simulink library "normalForce_ul"  (R2020a)
settings: Solver=VariableStepAuto  StartTime=0.0  StopTime=10.0  RelTol=1e-3
undefined symbols (not defined in the file): Veh
libraries: simulink x2, vrlib x1
settings Model: Creator=John Jr  LastModifiedBy=John Jr

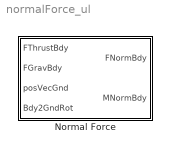
== system normalForce_ul ==
  Normal Force : Subsystem
      mask Display:
      | patch([0 1 1 0], [0 0 1 1],[.8 1 1])
      | 
      | port_label('input',1,'\fontname{Cambria Math}FThrustBdy','texmode','on')
      | port_label('input',2,'\fontname{Cambria Math}FGravBdy','texmode','on')
      | port_label('input',3,'\fontname{Cambria Math}posVecGnd','texmode','on')
      | port_label('input',4,'\fontname{Cambria Math}Bdy2GndRot','texmode','on')
      | 
      | port_label('output',1,'\fontname{Cambria Math}FNormBdy','texmode','on')
      | port_label('output',2,'\fontname{Cambria Math}MNormBdy','texmode','on')

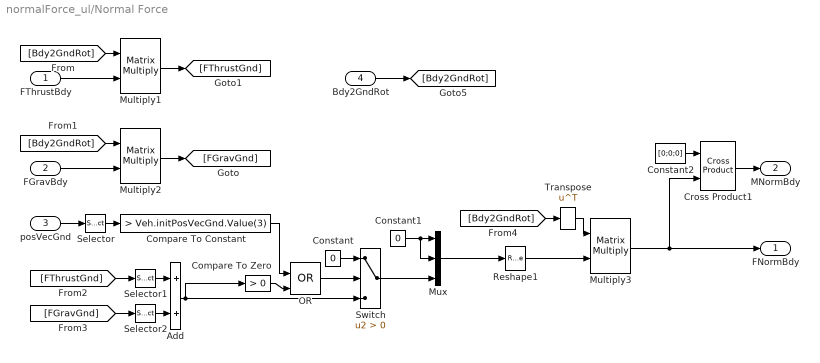
== system normalForce_ul/Normal Force ==
  FThrustBdy : Inport
  FGravBdy : Inport  Port=2
  posVecGnd : Inport  Port=3
  Bdy2GndRot : Inport  Port=4
  Add : Sum
  Compare To Constant : simulink/Logic and Bit Operations/Compare To Constant  relop=>  const=Veh.initPosVecGnd.Value(3)  OutDataTypeStr=boolean
  Compare To Zero : simulink/Logic and Bit Operations/Compare To Zero  relop=>  OutDataTypeStr=boolean
  Constant : Constant  Value=0
  Constant1 : Constant  Value=0
  Constant2 : Constant  Value=[0;0;0]
  Cross Product1 : vrlib/Utilities/Cross Product
  Multiply1 : Product  Multiplication=Matrix(*)
  Multiply2 : Product  Multiplication=Matrix(*)
  Multiply3 : Product  Multiplication=Matrix(*)
  Mux : Mux  Inputs=3
  OR : Logic  Operator=OR  IconShape=distinctive  AllPortsSameDT=off  OutDataTypeStr=boolean
  Reshape1 : Reshape  OutputDimensionality=Column vector (2-D)
  Selector : Selector  InputPortWidth=3  IndexOptions=Index vector (dialog)  Indices=3  OutputSizes=1
  Selector1 : Selector  InputPortWidth=3  IndexOptions=Index vector (dialog)  Indices=3  OutputSizes=1
  Selector2 : Selector  InputPortWidth=3  IndexOptions=Index vector (dialog)  Indices=3  OutputSizes=1
  Switch : Switch  Criteria=u2 > Threshold
  Transpose : Math  Operator=transpose  SignedPower=on  SaturateOnIntegerOverflow=on
  FNormBdy : Outport  VectorParamsAs1DForOutWhenUnconnected=off
  MNormBdy : Outport  Port=2  VectorParamsAs1DForOutWhenUnconnected=off
  wires:
  Selector/1 -> Compare To Constant/1
  Compare To Zero/1 -> OR/2
  Add/1 -> Compare To Zero/1, Switch/3
  OR/1 -> Switch/2
  Constant/1 -> Switch/1
  posVecGnd/1 -> Selector/1
  Bdy2GndRot/1 -> [Bdy2GndRot]
  FThrustBdy/1 -> Multiply1/2
  FGravBdy/1 -> Multiply2/2
  [Bdy2GndRot] -> Multiply1/1
  [Bdy2GndRot] -> Multiply2/1
  Multiply1/1 -> [FThrustGnd]
  Multiply2/1 -> [FGravGnd]
  [FThrustGnd] -> Selector1/1
  Selector1/1 -> Add/1
  [FGravGnd] -> Selector2/1
  Selector2/1 -> Add/2
  Constant2/1 -> Cross Product1/1
  Cross Product1/1 -> MNormBdy/1
  [Bdy2GndRot] -> Transpose/1
  Reshape1/1 -> Multiply3/2
  Transpose/1 -> Multiply3/1
  Multiply3/1 -> Cross Product1/2, FNormBdy/1
  Switch/1 -> Mux/3
  Constant1/1 -> Mux/2, Mux/1
  Mux/1 -> Reshape1/1
  Compare To Constant/1 -> OR/1
